simulink model "simscape_3dof"  (R2024a)
settings: Solver=ode45  StartTime=0.0  StopTime=20  FixedStep=1e-4  RelTol=1e-8  AbsTol=1e-10
values from neighbouring files (symbols this model uses):
  N = length(t)    [run_NE_ForwardDynamics.m]
undefined symbols (not defined in the file or in its folder): dq_IC_dps, X, Y, Z
libraries: nesl_utility x13, sm_lib x10
settings Model: Creator=91810  LastModifiedBy=91810

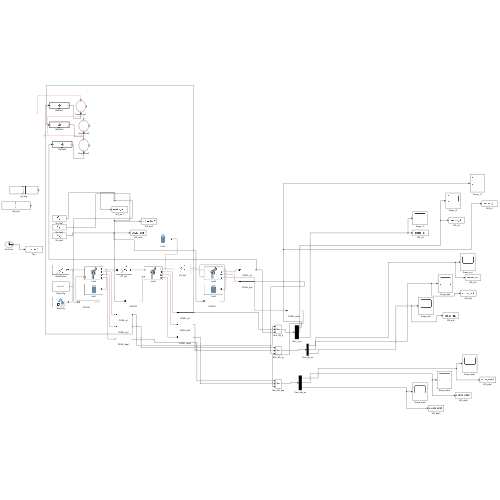
[thumbnail: Simulink's stored preview of the top-level diagram]
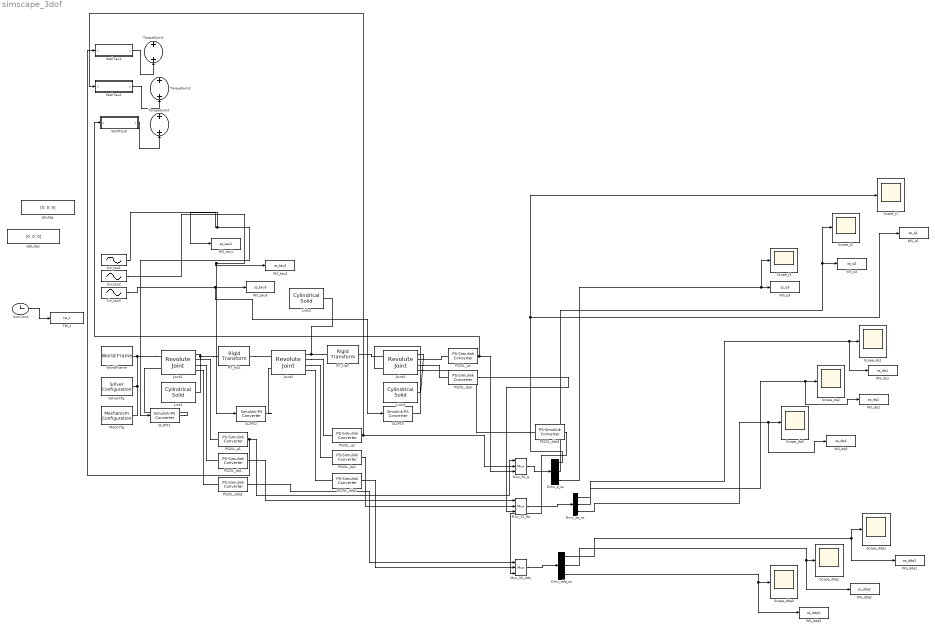
== system simscape_3dof ==
  Dmx_ddq_ss : Demux  Outputs=3
  Dmx_dq_ss : Demux  Outputs=3
  Dmx_q_ss : Demux  Outputs=3
  Joint1 : sm_lib/Joints/Revolute Joint  JointMode=Normal  CompositeWrenchDir=FollowerOnBase  CompositeWrenchFrame=BaseFrame  SenseConstraintForce=off  SenseConstraintTorque=off  SenseTotalForce=off  SenseTotalTorque=off  PositionTargetSpecify=on  PositionTargetPriority=High  PositionTargetValue=-90  PositionTargetValueUnits=deg  VelocityTargetSpecify=off  VelocityTargetPriority=High  VelocityTargetValue=dq_IC_dps(1)  VelocityTargetValueUnits=deg/s  EquilibriumPosition=0  EquilibriumPositionUnits=deg  SpringStiffness=0  SpringStiffnessUnits=N*m/deg  DampingCoefficient=0  DampingCoefficientUnits=N*m/(deg/s)  LowerLimitSpecify=off  LowerLimitBound=-90  LowerLimitBoundUnits=deg  LowerLimitStiffness=1e4  LowerLimitStiffnessUnits=N*m/deg  LowerLimitDamping=10  LowerLimitDampingUnits=N*m/(deg/s)  LowerLimitTransitionRegionWidth=0.1  LowerLimitTransitionRegionWidthUnits=deg  UpperLimitSpecify=off  UpperLimitBound=90  UpperLimitBoundUnits=deg  UpperLimitStiffness=1e4  UpperLimitStiffnessUnits=N*m/deg  UpperLimitDamping=10  UpperLimitDampingUnits=N*m/(deg/s)  UpperLimitTransitionRegionWidth=0.1  UpperLimitTransitionRegionWidthUnits=deg  TorqueActuationMode=InputTorque  MotionActuationMode=ComputedMotion  SensePosition=on  SenseVelocity=on  SenseAcceleration=on  SenseTorqueForce=off  SenseLowerLimitTorqueForce=off  SenseUpperLimitTorqueForce=off
  Joint2 : sm_lib/Joints/Revolute Joint  JointMode=Normal  CompositeWrenchDir=FollowerOnBase  CompositeWrenchFrame=BaseFrame  SenseConstraintForce=off  SenseConstraintTorque=off  SenseTotalForce=off  SenseTotalTorque=off  PositionTargetSpecify=on  PositionTargetPriority=High  PositionTargetValue=0  PositionTargetValueUnits=deg  VelocityTargetSpecify=off  VelocityTargetPriority=High  VelocityTargetValue=dq_IC_dps(2)  VelocityTargetValueUnits=deg/s  EquilibriumPosition=0  EquilibriumPositionUnits=deg  SpringStiffness=0  SpringStiffnessUnits=N*m/deg  DampingCoefficient=0  DampingCoefficientUnits=N*m/(deg/s)  LowerLimitSpecify=off  LowerLimitBound=-90  LowerLimitBoundUnits=deg  LowerLimitStiffness=1e4  LowerLimitStiffnessUnits=N*m/deg  LowerLimitDamping=10  LowerLimitDampingUnits=N*m/(deg/s)  LowerLimitTransitionRegionWidth=0.1  LowerLimitTransitionRegionWidthUnits=deg  UpperLimitSpecify=off  UpperLimitBound=90  UpperLimitBoundUnits=deg  UpperLimitStiffness=1e4  UpperLimitStiffnessUnits=N*m/deg  UpperLimitDamping=10  UpperLimitDampingUnits=N*m/(deg/s)  UpperLimitTransitionRegionWidth=0.1  UpperLimitTransitionRegionWidthUnits=deg  TorqueActuationMode=InputTorque  MotionActuationMode=ComputedMotion  SensePosition=on  SenseVelocity=on  SenseAcceleration=on  SenseTorqueForce=off  SenseLowerLimitTorqueForce=off  SenseUpperLimitTorqueForce=off
  Joint3 : sm_lib/Joints/Revolute Joint  JointMode=Normal  CompositeWrenchDir=FollowerOnBase  CompositeWrenchFrame=BaseFrame  SenseConstraintForce=off  SenseConstraintTorque=off  SenseTotalForce=off  SenseTotalTorque=off  PositionTargetSpecify=on  PositionTargetPriority=High  PositionTargetValue=0  PositionTargetValueUnits=deg  VelocityTargetSpecify=off  VelocityTargetPriority=High  VelocityTargetValue=dq_IC_dps(3)  VelocityTargetValueUnits=deg/s  EquilibriumPosition=0  EquilibriumPositionUnits=deg  SpringStiffness=0  SpringStiffnessUnits=N*m/deg  DampingCoefficient=0  DampingCoefficientUnits=N*m/(deg/s)  LowerLimitSpecify=off  LowerLimitBound=-90  LowerLimitBoundUnits=deg  LowerLimitStiffness=1e4  LowerLimitStiffnessUnits=N*m/deg  LowerLimitDamping=10  LowerLimitDampingUnits=N*m/(deg/s)  LowerLimitTransitionRegionWidth=0.1  LowerLimitTransitionRegionWidthUnits=deg  UpperLimitSpecify=off  UpperLimitBound=90  UpperLimitBoundUnits=deg  UpperLimitStiffness=1e4  UpperLimitStiffnessUnits=N*m/deg  UpperLimitDamping=10  UpperLimitDampingUnits=N*m/(deg/s)  UpperLimitTransitionRegionWidth=0.1  UpperLimitTransitionRegionWidthUnits=deg  TorqueActuationMode=InputTorque  MotionActuationMode=ComputedMotion  SensePosition=on  SenseVelocity=on  SenseAcceleration=on  SenseTorqueForce=off  SenseLowerLimitTorqueForce=off  SenseUpperLimitTorqueForce=off
  Link1 : sm_lib/Body Elements/Cylindrical Solid  CylinderRadius=0.06  CylinderRadiusUnits=m  CylinderLength=0.5  CylinderLengthUnits=m  ExportEntireGeometry=off  InertiaType=Custom  BasedOnType=Mass  Density=1000  DensityUnits=kg/m^3  Mass=2  MassUnits=kg  CenterOfMass=[0.2500 0 0]  CenterOfMassUnits=m  MomentsOfInertia=[0.00360000 0.04346667 0.04346667]  MomentsOfInertiaUnits=kg*m^2  ProductsOfInertia=[0 0 0]  ProductsOfInertiaUnits=kg*m^2  GraphicType=FromGeometry  MarkerShape=Sphere  MarkerSize=10  GraphicVisPropType=SimpleVisualProperties  GraphicDiffuseColor=[0.5 0.5 0.5]  GraphicOpacity=1  GraphicSpecularColor=[0.5 0.5 0.5 1.0]  GraphicAmbientColor=[0.15 0.15 0.15 1.0]  GraphicEmissiveColor=[0.0 0.0 0.0 1.0]  GraphicShininess=75  DoExposeReferenceFrame=on  SerializedFrames=<Frames/>
  Link2 : sm_lib/Body Elements/Cylindrical Solid  CylinderRadius=0.05  CylinderRadiusUnits=m  CylinderLength=0.4  CylinderLengthUnits=m  ExportEntireGeometry=off  InertiaType=Custom  BasedOnType=Mass  Density=1000  DensityUnits=kg/m^3  Mass=1.5  MassUnits=kg  CenterOfMass=[0.2000 0 0]  CenterOfMassUnits=m  MomentsOfInertia=[0.001875 0.0209375 0.0209375]  MomentsOfInertiaUnits=kg*m^2  ProductsOfInertia=[0 0 0]  ProductsOfInertiaUnits=kg*m^2  GraphicType=FromGeometry  MarkerShape=Sphere  MarkerSize=10  GraphicVisPropType=SimpleVisualProperties  GraphicDiffuseColor=[0.5 0.5 0.5]  GraphicOpacity=1  GraphicSpecularColor=[0.5 0.5 0.5 1.0]  GraphicAmbientColor=[0.15 0.15 0.15 1.0]  GraphicEmissiveColor=[0.0 0.0 0.0 1.0]  GraphicShininess=75  DoExposeReferenceFrame=on  SerializedFrames=<Frames/>
  Link3 : sm_lib/Body Elements/Cylindrical Solid  CylinderRadius=0.04  CylinderRadiusUnits=m  CylinderLength=0.3  CylinderLengthUnits=m  ExportEntireGeometry=off  InertiaType=Custom  BasedOnType=Mass  Density=1000  DensityUnits=kg/m^3  Mass=1  MassUnits=kg  CenterOfMass=[0.1500 0 0]  CenterOfMassUnits=m  MomentsOfInertia=[0.00080000 0.00790000 0.00790000]  MomentsOfInertiaUnits=kg*m^2  ProductsOfInertia=[0 0 0]  ProductsOfInertiaUnits=kg*m^2  GraphicType=FromGeometry  MarkerShape=Sphere  MarkerSize=10  GraphicVisPropType=SimpleVisualProperties  GraphicDiffuseColor=[0.5 0.5 0.5]  GraphicOpacity=1  GraphicSpecularColor=[0.5 0.5 0.5 1.0]  GraphicAmbientColor=[0.15 0.15 0.15 1.0]  GraphicEmissiveColor=[0.0 0.0 0.0 1.0]  GraphicShininess=75  DoExposeReferenceFrame=on  SerializedFrames=<Frames/>
  MechCfg : sm_lib/Utilities/Mechanism Configuration  UniformGravity=Constant  GravityVector=[0 -9.81 0]  GravityVectorUnits=m/s^2  LinearizationDelta=0.001  JointModeTransitionNonlinearIterations=2
  Mux_SS_ddq : Mux  Inputs=3
  Mux_SS_dq : Mux  Inputs=3
  Mux_SS_q : Mux  Inputs=3
  PS2SL_ddq1 : nesl_utility/PS-Simulink Converter  PhysicalDomain=network_engine_domain  SubClassName=ps_output  LeftPortType=input  RightPortType=output  PseudoPeriodic=off  Frequencies=[]  VectorFormat=inherit  Unit=inherit  AffineConversion=off
  PS2SL_ddq2 : nesl_utility/PS-Simulink Converter  PhysicalDomain=network_engine_domain  SubClassName=ps_output  LeftPortType=input  RightPortType=output  PseudoPeriodic=off  Frequencies=[]  VectorFormat=inherit  Unit=inherit  AffineConversion=off
  PS2SL_ddq3 : nesl_utility/PS-Simulink Converter  PhysicalDomain=network_engine_domain  SubClassName=ps_output  LeftPortType=input  RightPortType=output  PseudoPeriodic=off  Frequencies=[]  VectorFormat=inherit  Unit=inherit  AffineConversion=off
  PS2SL_dq1 : nesl_utility/PS-Simulink Converter  PhysicalDomain=network_engine_domain  SubClassName=ps_output  LeftPortType=input  RightPortType=output  PseudoPeriodic=off  Frequencies=[]  VectorFormat=inherit  Unit=inherit  AffineConversion=off
  PS2SL_dq2 : nesl_utility/PS-Simulink Converter  PhysicalDomain=network_engine_domain  SubClassName=ps_output  LeftPortType=input  RightPortType=output  PseudoPeriodic=off  Frequencies=[]  VectorFormat=inherit  Unit=inherit  AffineConversion=off
  PS2SL_dq3 : nesl_utility/PS-Simulink Converter  PhysicalDomain=network_engine_domain  SubClassName=ps_output  LeftPortType=input  RightPortType=output  PseudoPeriodic=off  Frequencies=[]  VectorFormat=inherit  Unit=inherit  AffineConversion=off
  PS2SL_q1 : nesl_utility/PS-Simulink Converter  PhysicalDomain=network_engine_domain  SubClassName=ps_output  LeftPortType=input  RightPortType=output  PseudoPeriodic=off  Frequencies=[]  VectorFormat=inherit  Unit=inherit  AffineConversion=off
  PS2SL_q2 : nesl_utility/PS-Simulink Converter  PhysicalDomain=network_engine_domain  SubClassName=ps_output  LeftPortType=input  RightPortType=output  PseudoPeriodic=off  Frequencies=[]  VectorFormat=inherit  Unit=inherit  AffineConversion=off
  PS2SL_q3 : nesl_utility/PS-Simulink Converter  PhysicalDomain=network_engine_domain  SubClassName=ps_output  LeftPortType=input  RightPortType=output  PseudoPeriodic=off  Frequencies=[]  VectorFormat=inherit  Unit=inherit  AffineConversion=off
  RT_tip1 : sm_lib/Frames and Transforms/Rigid Transform  RotationMethod=None  FollAlignAxisA=+X  BaseAlignAxisA=+Y  FollAlignAxisB=+Y  BaseAlignAxisB=+Z  RotationStandardAxis=+Z  RotationAngle=0  RotationAngleUnits=deg  RotationArbitraryAxis=[0 0 1]  RotationSequenceAxes=FollowerAxes  RotationSequence=XYX  RotationSequenceAngles=[0 0 0]  RotationSequenceAnglesUnits=deg  RotationMatrix=[1 0 0;0 1 0;0 0 1]  Quaternion=[1 0 0 0]  TranslationMethod=Cartesian  TranslationCartesianOffset=[0.5000 0 0]  TranslationCartesianOffsetUnits=m  TranslationStandardAxis=+Z  TranslationStandardOffset=0  TranslationStandardOffsetUnits=m  TranslationROffset=0  TranslationROffsetUnits=m  TranslationThetaOffset=0  TranslationThetaOffsetUnits=deg  TranslationZOffset=0  TranslationZOffsetUnits=m
  RT_tip2 : sm_lib/Frames and Transforms/Rigid Transform  RotationMethod=None  FollAlignAxisA=+X  BaseAlignAxisA=+Y  FollAlignAxisB=+Y  BaseAlignAxisB=+Z  RotationStandardAxis=+Z  RotationAngle=0  RotationAngleUnits=deg  RotationArbitraryAxis=[0 0 1]  RotationSequenceAxes=FollowerAxes  RotationSequence=XYX  RotationSequenceAngles=[0 0 0]  RotationSequenceAnglesUnits=deg  RotationMatrix=[1 0 0;0 1 0;0 0 1]  Quaternion=[1 0 0 0]  TranslationMethod=Cartesian  TranslationCartesianOffset=[0.4000 0 0]  TranslationCartesianOffsetUnits=m  TranslationStandardAxis=+Z  TranslationStandardOffset=0  TranslationStandardOffsetUnits=m  TranslationROffset=0  TranslationROffsetUnits=m  TranslationThetaOffset=0  TranslationThetaOffsetUnits=deg  TranslationZOffset=0  TranslationZOffsetUnits=m
  SL2PS1 : nesl_utility/Simulink-PS Converter  PhysicalDomain=network_engine_domain  SubClassName=ps_input  LeftPortType=input  RightPortType=output  PseudoPeriodic=off  Frequencies=[]  NoiseDistribution=none  NoiseParameters=[]  Unit=1  AffineConversion=off  FilteringAndDerivatives=provide  SimscapeFilterOrder=1  InputFilterTimeConstant=0.001  UdotUserProvided=0
  SL2PS2 : nesl_utility/Simulink-PS Converter  PhysicalDomain=network_engine_domain  SubClassName=ps_input  LeftPortType=input  RightPortType=output  PseudoPeriodic=off  Frequencies=[]  NoiseDistribution=none  NoiseParameters=[]  Unit=1  AffineConversion=off  FilteringAndDerivatives=provide  SimscapeFilterOrder=1  InputFilterTimeConstant=0.001  UdotUserProvided=0
  SL2PS3 : nesl_utility/Simulink-PS Converter  PhysicalDomain=network_engine_domain  SubClassName=ps_input  LeftPortType=input  RightPortType=output  PseudoPeriodic=off  Frequencies=[]  NoiseDistribution=none  NoiseParameters=[]  Unit=1  AffineConversion=off  FilteringAndDerivatives=provide  SimscapeFilterOrder=1  InputFilterTimeConstant=0.001  UdotUserProvided=0
  Scope_J1 : Scope
  Scope_J2 : Scope
  Scope_J3 : Scope
  Scope_ddq1 : Scope
  Scope_ddq2 : Scope
  Scope_ddq3 : Scope
  Scope_dq1 : Scope
  Scope_dq2 : Scope
  Scope_dq3 : Scope
  SimClock : Clock
  Sin_tau1 : Sin  Amplitude=3  Frequency=0.3  SampleTime=0
  Sin_tau2 : Sin  Frequency=0.5  Phase=0.785398163397448  SampleTime=0
  Sin_tau3 : Sin  Amplitude=0.3  Frequency=0.7  Phase=1.047197551196598  SampleTime=0
  SolverCfg : nesl_utility/Solver Configuration  PhysicalDomain=network_engine_domain  SubClassName=solver  LeftPortType=input  RightPortType=generic  Tones=[]  Harmonics=[]  SimulateNoise=off  Profile=off  UseLocalSampling=off  EnableSwitchedLinearOptims=on  FrequencyDomain=off  UseCCode=off  RelTol=0.001  AbsTol=0.001  MinStep=1e-09  ToWorkspace=off  RevertToSquareIcSolve=off  NumHomotopyIterations=100  PhasorMode=off  PhasorModeNumHarmonics=1  ConsistencySolver=NEWTON_XTOL_AFTER_FTOL  IndexReductionMethod=DerivativeReplacement  DoDC=off  ResidualTolerance=1e-09  ConsistencyTolSource=GLOBAL  ConsistencyAbsTol=0.001  ConsistencyRelTol=0.001  ConsistencyTolFactor=0.001  UseLocalSolver=off  LocalSolverChoice=NE_BACKWARD_EULER_ADVANCER  ResolveIndetEquations=on  FunctionEvalNumThread=1  LocalSolverSampleTime=0.001  DoFixedCost=off  MaxNonlinIter=3  MaxModeIter=2  ComputeImpulses=off  ImpulseIterations=2  LinearAlgebra=auto  LinearAlgebraNumThread=0  EquationFormulation=NE_TIME_EF  DelaysMemoryBudget=1024  AutomaticFiltering=on  FilteringTimeConstant=0.001  PartitionStorageMethod=AS_NEEDED  PartitionMemoryBudget=1024  PartitionMethod=ROBUST  MultibodyUseLocalSolver=off  MultibodyLocalSolverChoice=ODE1  MultibodyLocalSolverSampleTime=0.001
  TW_t : ToWorkspace  VariableName=tw_t  SampleTime=0.0001
  TorqueSum1 : Sum
  TorqueSum2 : Sum
  TorqueSum3 : Sum
  WS_ddq1 : ToWorkspace  VariableName=ss_ddq1  SampleTime=-1
  WS_ddq2 : ToWorkspace  VariableName=ss_ddq2  SampleTime=-1
  WS_ddq3 : ToWorkspace  VariableName=ss_ddq3  SampleTime=-1
  WS_dq1 : ToWorkspace  VariableName=ss_dq1  SampleTime=-1
  WS_dq2 : ToWorkspace  VariableName=ss_dq2  SampleTime=-1
  WS_dq3 : ToWorkspace  VariableName=ss_dq3  SampleTime=-1
  WS_q1 : ToWorkspace  VariableName=ss_q1  SampleTime=-1
  WS_q2 : ToWorkspace  VariableName=ss_q2  SampleTime=-1
  WS_q3 : ToWorkspace  VariableName=ss_q3  SampleTime=-1
  WS_tau1 : ToWorkspace  VariableName=ss_tau1  SampleTime=-1
  WS_tau2 : ToWorkspace  VariableName=ss_tau2  SampleTime=-1
  WS_tau3 : ToWorkspace  VariableName=ss_tau3  SampleTime=-1
  WallTau1 : MATLAB Function  TreatAsAtomicUnit=on
  WallTau2 : MATLAB Function  TreatAsAtomicUnit=on
  WallTau3 : MATLAB Function  TreatAsAtomicUnit=on
  WorldFrame : sm_lib/Frames and Transforms/World Frame
  dq0_dps : Constant  Value=[0; 0; 0]  VectorParams1D=off
  q0_deg : Constant  Value=[0; 0; 0]  VectorParams1D=off
  wires:
  Dmx_ddq_ss/1 -> WS_ddq1/1, Scope_ddq1/1
  SimClock/1 -> TW_t/1
  Dmx_ddq_ss/3 -> WS_ddq3/1, Scope_ddq3/1
  Dmx_ddq_ss/2 -> WS_ddq2/1, Scope_ddq2/1
  Dmx_dq_ss/3 -> WS_dq3/1, Scope_dq3/1
  Dmx_q_ss/3 -> WS_q3/1, Scope_J3/1
  PS2SL_q1/1 -> Mux_SS_q/1, WallTau1/1(u)
  Mux_SS_ddq/1 -> Dmx_ddq_ss/1
  Dmx_dq_ss/1 -> WS_dq1/1, Scope_dq1/1
  PS2SL_ddq2/1 -> Mux_SS_ddq/2
  Mux_SS_dq/1 -> Dmx_dq_ss/1
  Dmx_q_ss/1 -> WS_q1/1, Scope_J1/1
  Mux_SS_q/1 -> Dmx_q_ss/1
  PS2SL_dq2/1 -> Mux_SS_dq/2
  PS2SL_q2/1 -> Mux_SS_q/2, WallTau2/1(u)
  Dmx_q_ss/2 -> Scope_J2/1, WS_q2/1
  PS2SL_dq3/1 -> Mux_SS_dq/3
  PS2SL_ddq3/1 -> Mux_SS_ddq/3
  PS2SL_q3/1 -> Mux_SS_q/3, WallTau3/1(u)
  Dmx_dq_ss/2 -> WS_dq2/1, Scope_dq2/1
  PS2SL_dq1/1 -> Mux_SS_dq/1
  PS2SL_ddq1/1 -> Mux_SS_ddq/1
  ? -> TorqueSum1/1
  WallTau1/1(y) -> TorqueSum1/2
  Sin_tau1/1 -> WS_tau1/1, SL2PS1/1
  ? -> TorqueSum2/1
  WallTau2/1(y) -> TorqueSum2/2
  Sin_tau2/1 -> WS_tau2/1, SL2PS2/1
  ? -> TorqueSum3/1
  WallTau3/1(y) -> TorqueSum3/2
  Sin_tau3/1 -> SL2PS3/1, WS_tau3/1
  connections:
  Joint1/LConn1 -- SolverCfg/RConn1 -- MechCfg/RConn1 -- WorldFrame/RConn1
  RT_tip1/LConn1 -- Link1/RConn1 -- Joint1/RConn1
  RT_tip2/LConn1 -- Link2/RConn1 -- Joint2/RConn1
  RT_tip1/RConn1 -- Joint2/LConn1
  SL2PS1/RConn1 -- Joint1/LConn2
  Joint1/RConn2 -- PS2SL_q1/LConn1
  Joint3/RConn4 -- PS2SL_ddq3/LConn1
  RT_tip2/RConn1 -- Joint3/LConn1
  Joint3/RConn1 -- Link3/RConn1
  Joint2/RConn3 -- PS2SL_dq2/LConn1
  Joint3/RConn2 -- PS2SL_q3/LConn1
  SL2PS2/RConn1 -- Joint2/LConn2
  Joint1/RConn3 -- PS2SL_dq1/LConn1
  Joint1/RConn4 -- PS2SL_ddq1/LConn1
  Joint2/RConn4 -- PS2SL_ddq2/LConn1
  Joint2/RConn2 -- PS2SL_q2/LConn1
  SL2PS3/RConn1 -- Joint3/LConn2
  Joint3/RConn3 -- PS2SL_dq3/LConn1

== matlab function simscape_3dof/WallTau1 ==
  data: u input; y output
function y = fcn(u)
y = 0;

== matlab function simscape_3dof/WallTau3 ==
  data: u input; y output
function y = fcn(u)
y = 0;

== matlab function simscape_3dof/WallTau2 ==
  data: u input; y output
function y = fcn(u)
y = 0;
